simulink model "flyback"  (R2023b)
settings: Solver=VariableStepAuto  StartTime=0.0  StopTime=0.01  RelTol=1e-3
libraries: spsMeanLib x2, spsSeriesRLCBranchLib x2, spsCurrentMeasurementLib x1, spsDCVoltageSourceLib x1, spsDiodeLib x1, spsIGBTLib x1, spsLinearTransformerLib x1, spsRMSLib x1, spsVoltageMeasurementLib x1, sps_lib x1
settings Model: Creator=sachi  LastModifiedBy=sachi

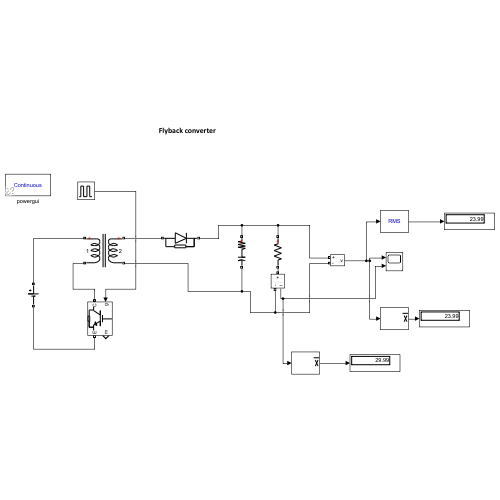
[thumbnail: Simulink's stored preview of the top-level diagram]
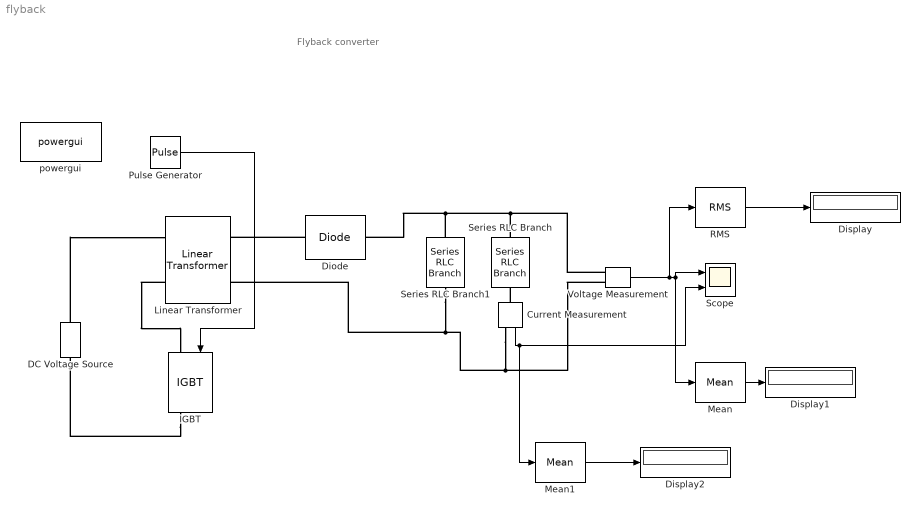
== system flyback ==
  note: Flyback converter
  Current Measurement : spsCurrentMeasurementLib/Current Measurement  PhasorSimulation=off  OutputType=Complex  PSBequivalent=0
  DC Voltage Source : spsDCVoltageSourceLib/DC Voltage Source  Amplitude=100  Measurements=None
  Diode : spsDiodeLib/Diode  Ron=0  Lon=0  Vf=0.7  IC=0  UseSnubber=0  Rs=500  Cs=250e-9  Measurements=off
  Display : Display
  Display1 : Display
  Display2 : Display
  IGBT : spsIGBTLib/IGBT  Ron=0  Lon=0  Vf=1.2  Tf=1e-6  Tt=2e-6  IC=0  Rs=1e5  Cs=inf  Measurements=on
  Linear Transformer : spsLinearTransformerLib/Linear Transformer  UNITS=pu  NominalPower=[ 1 1]  winding1=[1 0 0]  winding2=[0.25 0 0]  ThreeWindings=off  winding3=[3.15e+05 1.6e-08 1.0667e-05]  RmLm=[2160.8 36015]  Measurements=None  DataType=off
  Mean : spsMeanLib/Mean  Freq=1000  Vinit=0  Ts=0
  Mean1 : spsMeanLib/Mean  Freq=1000  Vinit=0  Ts=0
  Pulse Generator : DiscretePulseGenerator  PulseType=Time based  Amplitude=10  Period=0.001  PulseWidth=50  VectorParams1D=off
  RMS : spsRMSLib/RMS  TrueRMS=on  Freq=1000  RMSInit=120  Ts=0
  Scope : Scope  NumInputPorts=2
  Series RLC Branch : spsSeriesRLCBranchLib/Series RLC Branch  LConnTagsString=__new0  RConnTagsString=__new0  BranchType=R  Resistance=0.8  Inductance=1e-3  SetiL0=off  InitialCurrent=0  Capacitance=1e-6  Setx0=off  InitialVoltage=0  Measurements=None
  Series RLC Branch1 : spsSeriesRLCBranchLib/Series RLC Branch  LConnTagsString=__new0  RConnTagsString=__new0  BranchType=RC  Resistance=1e-4  Inductance=1e-3  SetiL0=off  InitialCurrent=0  Capacitance=1  Setx0=off  InitialVoltage=0  Measurements=None
  Voltage Measurement : spsVoltageMeasurementLib/Voltage Measurement  PhasorSimulation=off  OutputType=Complex  PSBequivalent=0
  powergui : sps_lib/powergui  Priority=1  SimulationMode=Continuous  SampleTime=50e-6  frequency=60  Iterations=50  frequencyindice=0  Pbase=100e6  ErrMax=1e-4  UnitsV=kV  UnitsW=MW  buscounter=0  FunctionMessages=off  echomessages=off  EnableUseOfTLC=off  CurrentSourceSwitches=off  DisableSnubberDevices=off  DisableRonSwitches=off  DisableVfSwitches=off  DisplayEquations=off  AutomaticDiscreteSolvers=off  SolverType=Tustin/Backward Euler (TBE)  Interpol=off  ExternalGateDelay=off  methode=off  Ts=100  x0status=blocks  SPID=on  SwTol=0  HookPort=off  NonlinearTolerance=1e-4  nMaxIteration=100  ContinueOnMaxIteration=off  RestoreLinks=warning  ResistiveCurrentMeasurement=off  Frange=[0:2:500]  Ylog=off  Xlog=on  ShowGrid=off  save=off  variable=ZData  structure=0  ZoomFFT=off  StartTime=0.0  cycles=1  DisplayStyle=1  fundamental=60  FreqAxis=off  MaxFrequency=1000  frequencyindicesteady=1  RmsSteady=1  display=off
  wires:
  Pulse Generator/1 -> IGBT/1
  Voltage Measurement/1 -> RMS/1, Mean/1, Scope/1
  RMS/1 -> Display/1
  Mean/1 -> Display1/1
  Current Measurement/1 -> Scope/2, Mean1/1
  Mean1/1 -> Display2/1
  connections:
  Diode/LConn1 -- Linear Transformer/RConn1
  DC Voltage Source/RConn1 -- Linear Transformer/LConn1
  Current Measurement/RConn1 -- Voltage Measurement/LConn2 -- Series RLC Branch1/RConn1 -- Linear Transformer/RConn2
  Current Measurement/LConn1 -- Series RLC Branch/RConn1
  Linear Transformer/LConn2 -- IGBT/LConn1
  IGBT/RConn1 -- DC Voltage Source/LConn1
  Voltage Measurement/LConn1 -- Series RLC Branch1/LConn1 -- Diode/RConn1 -- Series RLC Branch/LConn1
